simulink model "transmitter"  (R2023b)
settings: Solver=VariableStepAuto  StartTime=0.0  StopTime=10.0  RelTol=1e-3
settings Model: Creator=grace  LastModifiedBy=grace

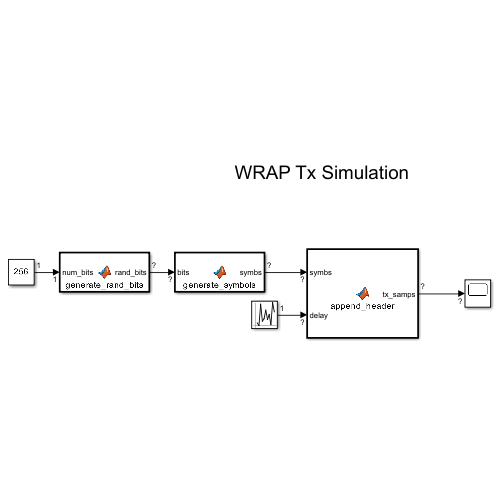
[thumbnail: Simulink's stored preview of the top-level diagram]
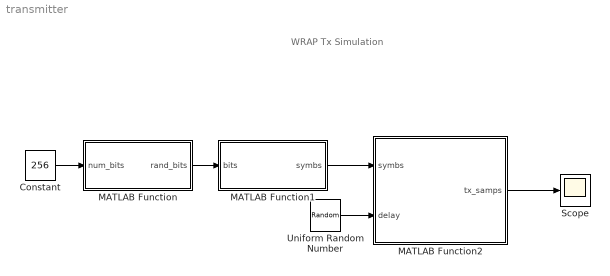
== system transmitter ==
  note: WRAP Tx Simulation
  Constant : Constant  Value=256
  MATLAB Function : MATLAB Function  TreatAsAtomicUnit=on
  MATLAB Function1 : MATLAB Function  TreatAsAtomicUnit=on
  MATLAB Function2 : MATLAB Function  TreatAsAtomicUnit=on
  Scope : Scope
  Uniform Random Number : UniformRandomNumber  Minimum=0  Maximum=100  SampleTime=0.1
  wires:
  MATLAB Function/1(rand_bits) -> MATLAB Function1/1(bits)
  Constant/1 -> MATLAB Function/1(num_bits)
  MATLAB Function1/1(symbs) -> MATLAB Function2/1(symbs)
  Uniform Random Number/1 -> MATLAB Function2/2(delay)
  MATLAB Function2/1(tx_samps) -> Scope/1

== matlab function transmitter/MATLAB Function ==
  data: num_bits input; rand_bits output int32 size=num_bits
function rand_bits = generate_rand_bits(num_bits)
rand_bits = randi([0,1],1,num_bits);
end

== matlab function transmitter/MATLAB Function2 ==
  data: tx_samps output; symbs input; delay input
function tx_samps = append_header(symbs, delay)
packet_header = repmat(constants.key,1,3);

packet = cat(2, packet_header, symbs);

num_packets = fix((constants.Ns-delay)/length(packet));
bits_remaining = rem((constants.Ns-delay),length(packet));

tx_symbs = [zeros(1, delay) repmat(packet,1,num_packets) zeros(1,bits_remaining)];
tx_samps = upsample(tx_symbs, constants.sps);
end

== matlab function transmitter/MATLAB Function1 ==
  data: bits input; symbs output
function symbs = generate_symbols(bits)
symbs = 2 * (bits - 0.5);
end
